simulink model "Problem_7"  (R2020a)
settings: Solver=VariableStepAuto  StartTime=0.0  StopTime=10.0  RelTol=1e-3
libraries: simulink x1
settings Model: Creator=Admin  LastModifiedBy=Admin

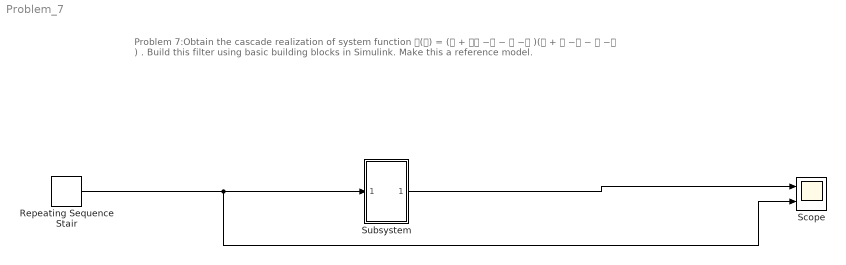
== system Problem_7 ==
  note: Problem 7:Obtain the cascade realization of system function
      | 𝐇(𝐳) = (𝟏 + 𝟐𝐳 −𝟏 − 𝐳 −𝟐 )(𝟏 + 𝐳 −𝟏 − 𝐳 −𝟐 ) .
      | Build this filter using basic building blocks in Simulink. Make this a reference model.
  Repeating Sequence Stair : simulink/Sources/Repeating Sequence Stair  OutValues=[3 1 4 2 1].'  tsamp=-1  OutMin=[]  OutMax=[]  OutDataTypeStr=double  OutputDataTypeScalingMode=double  OutDataType=fixdt(0,8)  ConRadixGroup=Best Precision: Vector-wise  OutScaling=2^-12
  Scope : Scope  NumInputPorts=2
  Subsystem : Subsystem
  wires:
  Repeating Sequence Stair/1 -> Subsystem/1(In1), Scope/2
  Subsystem/1(Out1) -> Scope/1

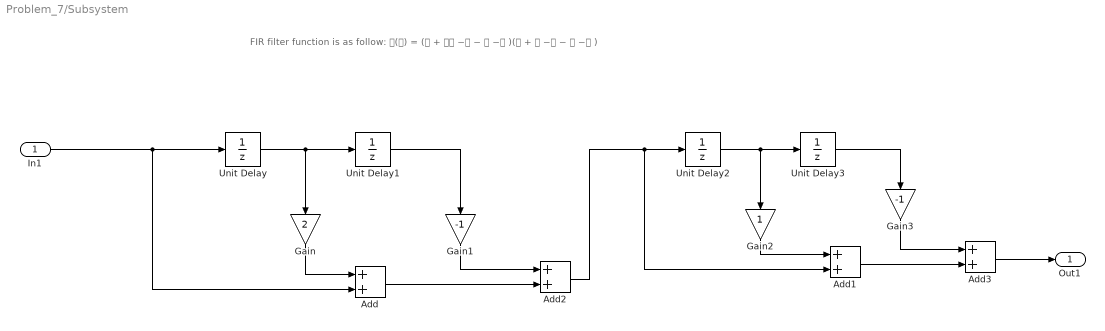
== system Problem_7/Subsystem ==
  note: FIR filter function is as follow:
      | 𝐇(𝐳) = (𝟏 + 𝟐𝐳 −𝟏 − 𝐳 −𝟐 )(𝟏 + 𝐳 −𝟏 − 𝐳 −𝟐 )
  In1 : Inport
  Add{,1..3} (4 alike) : Sum
  Gain : Gain  Gain=2
  Gain1 : Gain  Gain=-1
  Gain2 : Gain
  Gain3 : Gain  Gain=-1
  Unit Delay{,1..3} (4 alike) : UnitDelay  SampleTime=-1  HasFrameUpgradeWarning=on
  Out1 : Outport
  wires:
  Unit Delay1/1 -> Gain1/1
  Add1/1 -> Add3/2
  Unit Delay2/1 -> Gain2/1, Unit Delay3/1
  In1/1 -> Unit Delay/1, Add/2
  Unit Delay3/1 -> Gain3/1
  Gain/1 -> Add/1
  Gain3/1 -> Add3/1
  Unit Delay/1 -> Unit Delay1/1, Gain/1
  Add2/1 -> Add1/2, Unit Delay2/1
  Gain1/1 -> Add2/1
  Add/1 -> Add2/2
  Gain2/1 -> Add1/1
  Add3/1 -> Out1/1
